simulink model "f16longiModel"  (R2014a)
settings: Solver=ode45  StartTime=0.0  StopTime=300  RelTol=1e-3
values from neighbouring files (symbols this model uses):
  A = [.770 .241 -.100 -.416 -.731 -1.053 -1.366 -1.646 -1.917 -2.120 -2.248 -2.229]    [cz.m]    (also in damping.m = [-.267 -.110  .308  1.34  2.08  2.91  2.76  2.05   1.5  1.49)
  C = eye(4)    [trimF16.m]
  D = zeros(4,2)    [trimF16.m]
undefined symbols (not defined in the file or in its folder): B
settings Model: Creator=raktim  LastModifiedBy=raktim
settings DataIOCC: SignalLoggingSaveFormat=ModelDataLogs
settings OptimizationCC: ExpressionDepthLimit=2147483647
settings DebuggingCC: UnderspecifiedInitializationDetection=Classic  FcnCallInpInsideContextMsg=UseLocalSettings  StateNameClashWarn=warning  InitInArrayFormatMsg=none
settings GRTTargetCC: CombineOutputUpdateFcns=off  GRTInterface=on

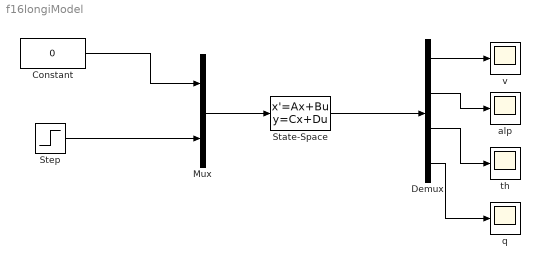
== system f16longiModel ==
  Constant : Constant  Value=0
  Demux : Demux
  Mux : Mux  Inputs=2
  State-Space : StateSpace  A=A  B=B  C=C  D=D  X0=0
  Step : Step  SampleTime=0
  alp : Scope
  q : Scope
      settings: SaveName=ScopeData3
  th : Scope
      settings: SaveName=ScopeData2
  v : Scope
  wires:
  Mux/1 -> State-Space/1
  Constant/1 -> Mux/1
  Step/1 -> Mux/2
  State-Space/1 -> Demux/1
  Demux/1 -> v/1
  Demux/2 -> alp/1
  Demux/3 -> th/1
  Demux/4 -> q/1
